simulink model "P1Ej4"  (R2022a)
settings: Solver=ode15s  StartTime=0.0  StopTime=10.0  RelTol=1e-3
settings Model: Creator=adrian.losada.alvare  LastModifiedBy=Adrian
settings DebuggingCC: UnconnectedInputMsg=warning  UnconnectedOutputMsg=warning  UnconnectedLineMsg=warning
settings RTWCC: DLArmComputeVersion=19.05

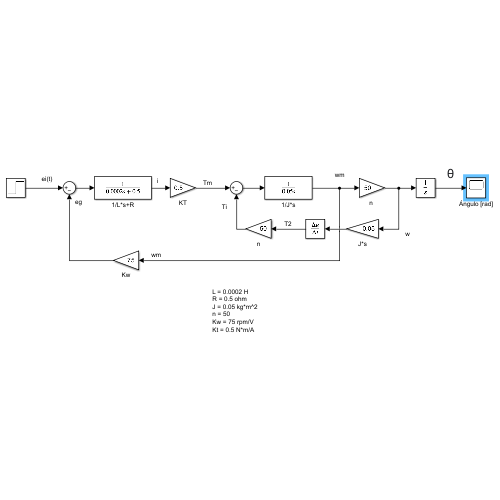
[thumbnail: Simulink's stored preview of the top-level diagram]
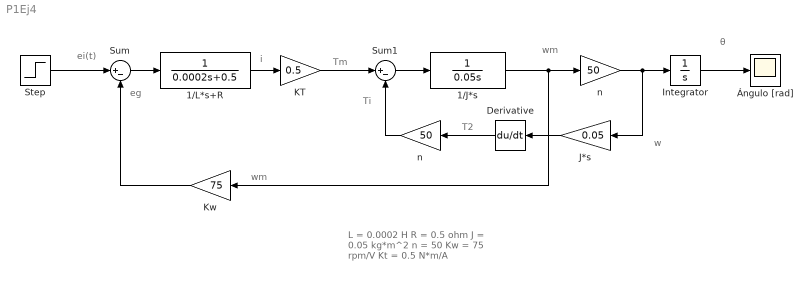
== system P1Ej4 ==
  note: θ
  note: ei(t)
  note: wm
  note: w
  note: T2
  note: Ti
  note: wm
  note: i
  note: Tm
  note: eg
  note: L = 0.0002 H
      | R = 0.5 ohm
      | J = 0.05 kg*m^2
      | n = 50
      | Kw = 75 rpm/V
      | Kt = 0.5 N*m/A
  1/J*s : TransferFcn  Denominator=[0.05 0]
  1/L*s+R : TransferFcn  Denominator=[0.0002 0.5]
  Derivative : Derivative
  Integrator : Integrator
  J*s : Gain  Gain=0.05
  KT : Gain  Gain=0.5
  Kw : Gain  Gain=75
  Step : Step  SampleTime=0
  Sum : Sum  Inputs=|+-
  Sum1 : Sum  Inputs=|+-
  n : Gain  Gain=50
  "n " : Gain  Gain=50
  Ángulo [rad] : Scope
  wires:
  Step/1 -> Sum/1
  Sum/1 -> 1/L*s+R/1
  1/L*s+R/1 -> KT/1
  Kw/1 -> Sum/2
  KT/1 -> Sum1/1
  Sum1/1 -> 1/J*s/1
  n/1 -> Sum1/2
  1/J*s/1 -> "n "/1, Kw/1
  "n "/1 -> J*s/1, Integrator/1
  Integrator/1 -> Ángulo [rad]/1
  Derivative/1 -> n/1
  J*s/1 -> Derivative/1
